simulink model "PneumaticDynamics"  (R2015a)
settings: Solver=ode45  StartTime=0.0  StopTime=120  RelTol=1e-3
InitFcn:
  | %Parameters
  | Patm = 101300; % Pascals
  | Psrc = Patm*2; % Pascals
  | Tamb = 293; %K - ambient temp
  | 
  | %Valve Geometry
  | stroke = 0.1; % m - stroke length
  | x0 = stroke / 2; % m -initial position
  | A = 0.080; % m2 - cap area
  | A_r = 0.02; % m2 - rod area
  | CapDeadSpace = 0.005; % meters - length past stroke
  | RodDeadSpace = 0.005; %meters - length past stroke
  | m = 3; % kg - rod/cap total mass
  | Cd = 0.8; % discharge coefficient
  | 
  | %Thermodynamic Values
  | k = 1.4; % specific heat ratio for air
  | R = 287; % J/Kg/K; % - specific gas constant for air
  | cp = 1012;% J/Kg/K; % - specific heat of air
  | 
  | %Fluid Flow Values
  | Pcr = 0.528; % choked flow ratio
  | C1 = sqrt(2*k/(R*(k-1))); % flow constant
  | C2 = sqrt( k/( R*((k+1)/2)^((k+1)/(k-1)) ) ); % flow cnst.
libraries: simulink x3
settings Model: Creator=Logan  LastModifiedBy=Logan

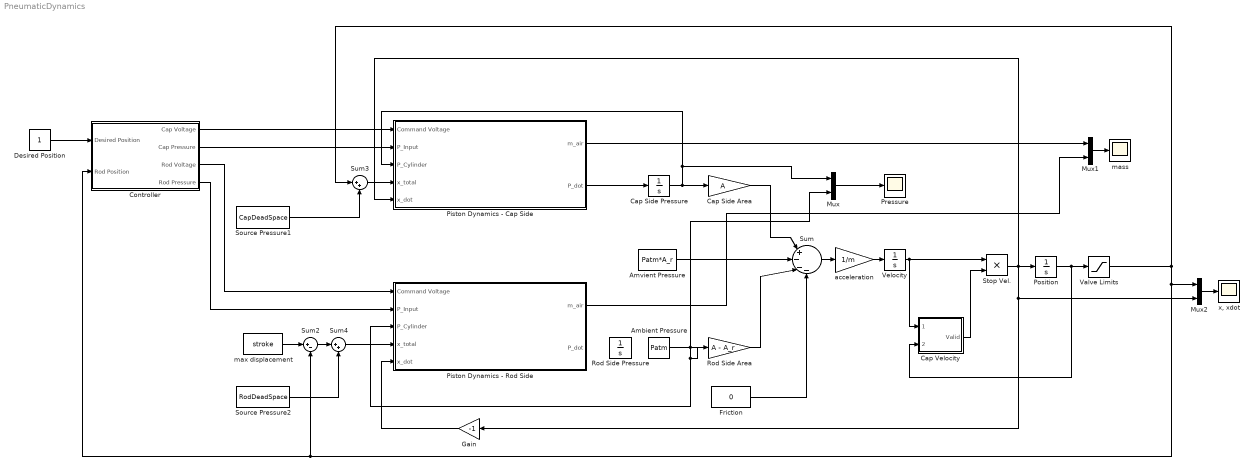
== system PneumaticDynamics ==
  Ambient Pressure : Constant  Value=Patm
  Amvient Pressure : Constant  Value=Patm*A_r
  Cap Side Area : Gain  Gain=A
  Cap Side Pressure : Integrator  InitialCondition=Patm  LimitOutput=on  LowerSaturationLimit=0
  Cap Velocity : Subsystem
  Controller : Subsystem
  Desired Position : Constant
  Friction : Constant  Value=0
  Gain : Gain  Gain=-1
  Mux : Mux  Inputs=2
  Mux1 : Mux  Inputs=2
  Mux2 : Mux  Inputs=2
  Piston Dynamics - Cap Side : Subsystem
  Piston Dynamics - Rod Side : Subsystem
  Position : Integrator  InitialCondition=x0
  Pressure : Scope
      settings: YMin=90000  YMax=155000
  Rod Side Area : Gain  Gain=A - A_r
  Rod Side Pressure : Integrator  InitialCondition=Patm  LimitOutput=on  LowerSaturationLimit=0
  Source Pressure1 : Constant  Value=CapDeadSpace
  Source Pressure2 : Constant  Value=RodDeadSpace
  Stop Vel. : Product
  Sum : Sum  Inputs=|+---
  Sum2 : Sum  Inputs=|+-
  Sum3 : Sum  Inputs=|++
  Sum4 : Sum  Inputs=|++
  Valve Limits : Saturate  UpperLimit=stroke  LowerLimit=0
  Velocity : Integrator
  acceleration : Gain  Gain=1/m
  mass : Scope
      settings: YMin=0.000275  YMax=0.000825
  max displacement : Constant  Value=stroke
  "x, xdot" : Scope
      settings: YMin=-0.0025  YMax=0.0525  SaveName=ScopeData2
  wires:
  Piston Dynamics - Cap Side/2(P_dot) -> Cap Side Pressure/1
  Cap Side Pressure/1 -> Mux/1, Piston Dynamics - Cap Side/3(P_Cylinder), Cap Side Area/1
  Ambient Pressure/1 -> Mux/2, Rod Side Area/1, Piston Dynamics - Rod Side/3(P_Cylinder)
  Cap Side Area/1 -> Sum/1
  Amvient Pressure/1 -> Sum/2
  Rod Side Area/1 -> Sum/3
  Friction/1 -> Sum/4
  Sum/1 -> acceleration/1
  acceleration/1 -> Velocity/1
  Position/1 -> Cap Velocity/2(Position), Valve Limits/1
  max displacement/1 -> Sum2/1
  Source Pressure1/1 -> Sum3/2
  Sum2/1 -> Sum4/1
  Sum4/1 -> Piston Dynamics - Rod Side/4(x_total)
  Source Pressure2/1 -> Sum4/2
  Sum3/1 -> Piston Dynamics - Cap Side/4(x_total)
  Valve Limits/1 -> Sum3/1, Controller/2(Rod Position), Sum2/2, Mux2/1
  Mux/1 -> Pressure/1
  Mux1/1 -> mass/1
  Piston Dynamics - Cap Side/1(m_air) -> Mux1/1
  Piston Dynamics - Rod Side/1(m_air) -> Mux1/2
  Mux2/1 -> "x, xdot"/1
  Stop Vel./1 -> Mux2/2, Gain/1, Position/1, Piston Dynamics - Cap Side/5(x_dot)
  Cap Velocity/1(Valid) -> Stop Vel./2
  Velocity/1 -> Stop Vel./1, Cap Velocity/1(Velocity)
  Desired Position/1 -> Controller/1(Desired Position)
  Controller/1(Cap Voltage) -> Piston Dynamics - Cap Side/1(Command Voltage)
  Controller/2(Cap Pressure) -> Piston Dynamics - Cap Side/2(P_Input)
  Controller/3(Rod Voltage) -> Piston Dynamics - Rod Side/1(Command Voltage)
  Controller/4(Rod Pressure) -> Piston Dynamics - Rod Side/2(P_Input)
  Gain/1 -> Piston Dynamics - Rod Side/5(x_dot)

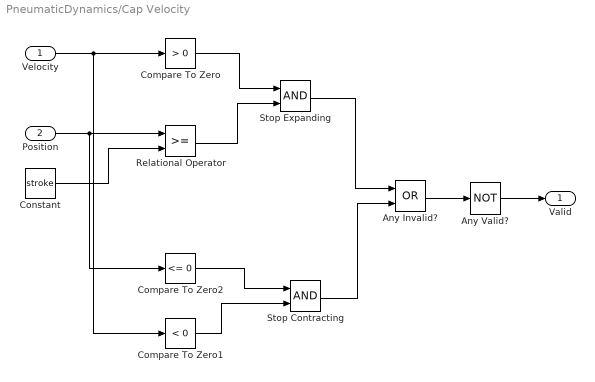
== system PneumaticDynamics/Cap Velocity ==
  Velocity : Inport
  Position : Inport  Port=2
  Any Invalid? : Logic  Operator=OR  AllPortsSameDT=off  OutDataTypeStr=boolean
  Any Valid? : Logic  Operator=NOT  AllPortsSameDT=off  OutDataTypeStr=boolean
  Compare To Zero : simulink/Logic and Bit Operations/Compare To Zero  relop=>  OutDataTypeStr=boolean
  Compare To Zero1 : simulink/Logic and Bit Operations/Compare To Zero  relop=<  OutDataTypeStr=boolean
  Compare To Zero2 : simulink/Logic and Bit Operations/Compare To Zero  relop=<=  OutDataTypeStr=boolean
  Constant : Constant  Value=stroke
  Relational Operator : RelationalOperator  OutDataTypeStr=boolean
  Stop Expanding : Logic  AllPortsSameDT=off  OutDataTypeStr=boolean
  Stop Contracting : Logic  AllPortsSameDT=off  OutDataTypeStr=boolean
  Valid : Outport
  wires:
  Position/1 -> Compare To Zero2/1, Relational Operator/1
  Constant/1 -> Relational Operator/2
  Velocity/1 -> Compare To Zero1/1, Compare To Zero/1
  Compare To Zero/1 -> Stop Expanding/1
  Relational Operator/1 -> Stop Expanding/2
  Compare To Zero2/1 -> Stop Contracting/1
  Compare To Zero1/1 -> Stop Contracting/2
  Stop Expanding/1 -> Any Invalid?/1
  Stop Contracting/1 -> Any Invalid?/2
  Any Invalid?/1 -> Any Valid?/1
  Any Valid?/1 -> Valid/1

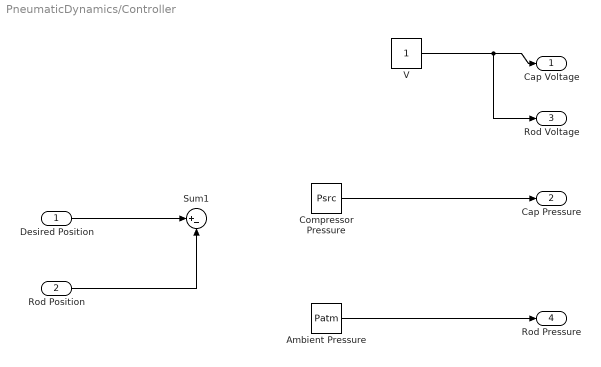
== system PneumaticDynamics/Controller ==
  Desired Position : Inport
  Rod Position : Inport  Port=2
  Ambient Pressure : Constant  Value=Patm
  Compressor Pressure : Constant  Value=Psrc
  Sum1 : Sum  Inputs=|+-
  V : Constant
  Cap Voltage : Outport
  Cap Pressure : Outport  Port=2
  Rod Voltage : Outport  Port=3
  Rod Pressure : Outport  Port=4
  wires:
  Rod Position/1 -> Sum1/2
  Desired Position/1 -> Sum1/1
  Compressor Pressure/1 -> Cap Pressure/1
  V/1 -> Rod Voltage/1, Cap Voltage/1
  Ambient Pressure/1 -> Rod Pressure/1

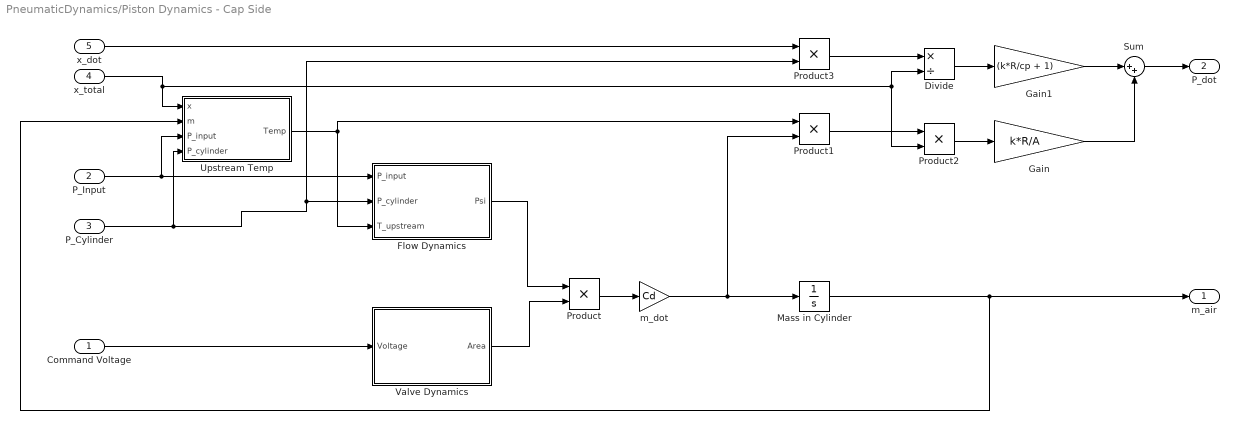
== system PneumaticDynamics/Piston Dynamics - Cap Side ==
  Command Voltage : Inport
  P_Input : Inport  Port=2
  P_Cylinder : Inport  Port=3
  x_total : Inport  Port=4
  x_dot : Inport  Port=5
  Divide : Product  Inputs=*/
  Flow Dynamics : Subsystem
  Gain : Gain  Gain=k*R/A
  Gain1 : Gain  Gain=(k*R/cp + 1)
  Mass in Cylinder : Integrator  InitialCondition=Patm*(x0*A)/R/Tamb
  Product{,1..3} (4 alike) : Product
  Sum : Sum  Inputs=|++
  Upstream Temp : Subsystem
  Valve Dynamics : Subsystem
  m_dot : Gain  Gain=Cd
  m_air : Outport
  P_dot : Outport  Port=2
  wires:
  Product1/1 -> Product2/1
  Product2/1 -> Gain/1
  m_dot/1 -> Mass in Cylinder/1, Product1/2
  Mass in Cylinder/1 -> m_air/1, Upstream Temp/2(m)
  Command Voltage/1 -> Valve Dynamics/1(Voltage)
  P_Input/1 -> Flow Dynamics/1(P_input), Upstream Temp/3(P_input)
  Product3/1 -> Divide/1
  Gain1/1 -> Sum/1
  Product/1 -> m_dot/1
  Divide/1 -> Gain1/1
  x_total/1 -> Product2/2, Divide/2, Upstream Temp/1(x)
  Gain/1 -> Sum/2
  x_dot/1 -> Product3/1
  Flow Dynamics/1(Psi) -> Product/1
  Valve Dynamics/1(Area) -> Product/2
  P_Cylinder/1 -> Flow Dynamics/2(P_cylinder), Product3/2, Upstream Temp/4(P_cylinder)
  Sum/1 -> P_dot/1
  Upstream Temp/1(Temp) -> Flow Dynamics/3(T_upstream), Product1/1

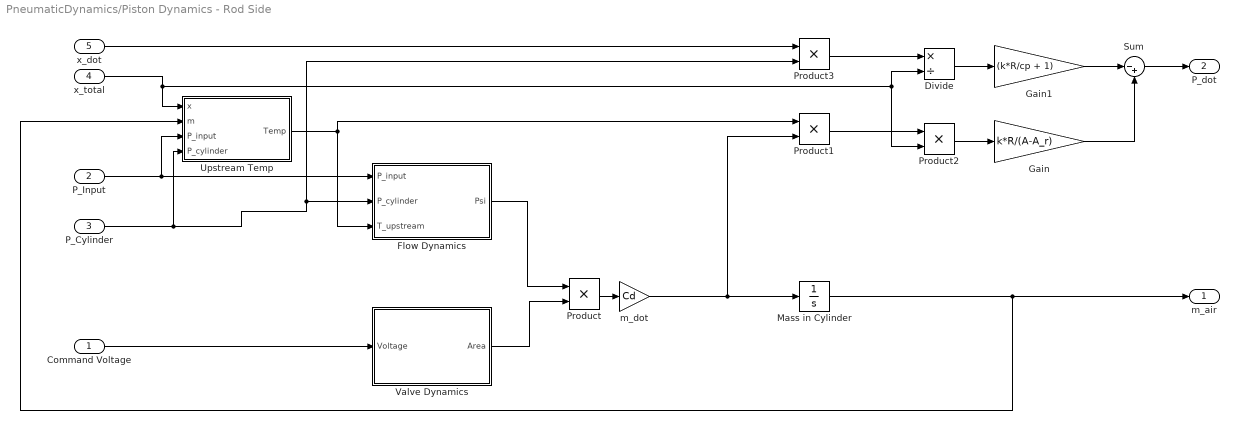
== system PneumaticDynamics/Piston Dynamics - Rod Side ==
  Command Voltage : Inport
  P_Input : Inport  Port=2
  P_Cylinder : Inport  Port=3
  x_total : Inport  Port=4
  x_dot : Inport  Port=5
  Divide : Product  Inputs=*/
  Flow Dynamics : Subsystem
  Gain : Gain  Gain=k*R/(A-A_r)
  Gain1 : Gain  Gain=(k*R/cp + 1)
  Mass in Cylinder : Integrator  InitialCondition=Patm*(x0*(A-A_r))/R/Tamb
  Product{,1..3} (4 alike) : Product
  Sum : Sum  Inputs=|-+
  Upstream Temp : Subsystem
  Valve Dynamics : Subsystem
  m_dot : Gain  Gain=Cd
  m_air : Outport
  P_dot : Outport  Port=2
  wires:
  Product1/1 -> Product2/1
  Product2/1 -> Gain/1
  m_dot/1 -> Mass in Cylinder/1, Product1/2
  Mass in Cylinder/1 -> Upstream Temp/2(m), m_air/1
  Command Voltage/1 -> Valve Dynamics/1(Voltage)
  P_Input/1 -> Flow Dynamics/1(P_input), Upstream Temp/3(P_input)
  Product3/1 -> Divide/1
  Gain1/1 -> Sum/1
  Product/1 -> m_dot/1
  Divide/1 -> Gain1/1
  x_total/1 -> Product2/2, Divide/2, Upstream Temp/1(x)
  Gain/1 -> Sum/2
  x_dot/1 -> Product3/1
  Flow Dynamics/1(Psi) -> Product/1
  Valve Dynamics/1(Area) -> Product/2
  P_Cylinder/1 -> Flow Dynamics/2(P_cylinder), Product3/2, Upstream Temp/4(P_cylinder)
  Sum/1 -> P_dot/1
  Upstream Temp/1(Temp) -> Flow Dynamics/3(T_upstream), Product1/1

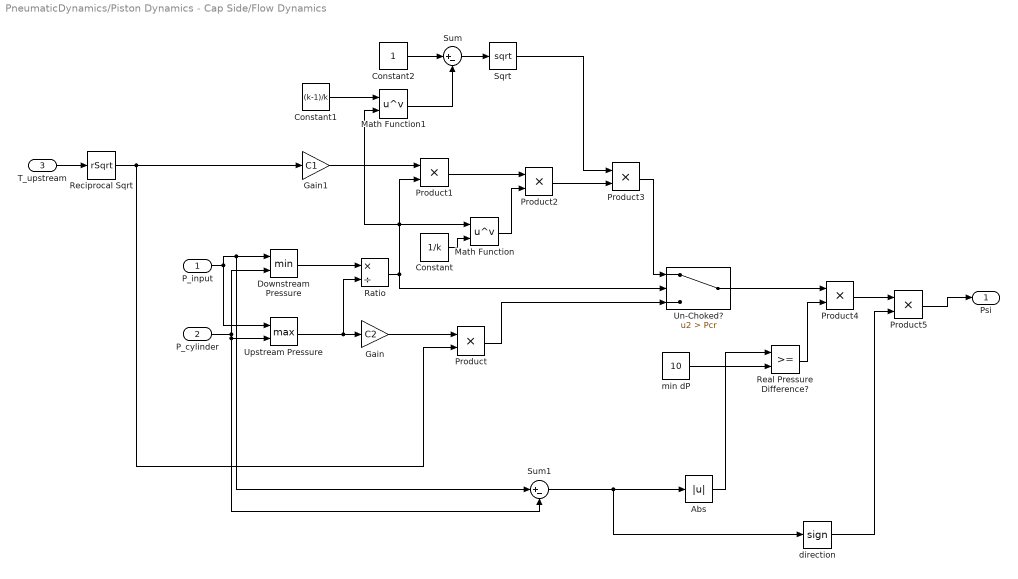
== system PneumaticDynamics/Piston Dynamics - Cap Side/Flow Dynamics ==
  P_input : Inport
  P_cylinder : Inport  Port=2
  T_upstream : Inport  Port=3
  Abs : Abs
  Constant : Constant  Value=1/k
  Constant1 : Constant  Value=(k-1)/k
  Constant2 : Constant
  Downstream Pressure : MinMax  Inputs=2
  Gain : Gain  Gain=C2
  Gain1 : Gain  Gain=C1
  Math Function : Math  Operator=pow  SaturateOnIntegerOverflow=on
  Math Function1 : Math  Operator=pow  SaturateOnIntegerOverflow=on
  Product{,1..5} (6 alike) : Product
  Ratio : Product  Inputs=*/
  Real Pressure Difference? : RelationalOperator  OutDataTypeStr=boolean  ZeroCross=off
  Reciprocal Sqrt : Sqrt  Operator=rSqrt  SaturateOnIntegerOverflow=on
  Sqrt : Sqrt  SaturateOnIntegerOverflow=on
  Sum : Sum  Inputs=|+-
  Sum1 : Sum  Inputs=|+-
  Un-Choked? : Switch  Criteria=u2 > Threshold  Threshold=Pcr  ZeroCross=off
  Upstream Pressure : MinMax  Function=max  Inputs=2
  direction : Signum
  min dP : Constant  Value=10
  Psi : Outport
  wires:
  P_input/1 -> Sum1/1, Downstream Pressure/1, Upstream Pressure/1
  P_cylinder/1 -> Downstream Pressure/2, Sum1/2, Upstream Pressure/2
  Ratio/1 -> Un-Choked?/2, Math Function1/2, Math Function/1, Product1/2
  T_upstream/1 -> Reciprocal Sqrt/1
  Gain/1 -> Product/1
  Reciprocal Sqrt/1 -> Gain1/1, Product/2
  Product/1 -> Un-Choked?/3
  Gain1/1 -> Product1/1
  Product1/1 -> Product2/1
  Constant/1 -> Math Function/2
  Math Function/1 -> Product2/2
  Constant2/1 -> Sum/1
  Math Function1/1 -> Sum/2
  Sum/1 -> Sqrt/1
  Product2/1 -> Product3/2
  Sqrt/1 -> Product3/1
  Constant1/1 -> Math Function1/1
  Product3/1 -> Un-Choked?/1
  Downstream Pressure/1 -> Ratio/1
  Upstream Pressure/1 -> Ratio/2, Gain/1
  Un-Choked?/1 -> Product4/1
  Sum1/1 -> direction/1, Abs/1
  Real Pressure Difference?/1 -> Product4/2
  Abs/1 -> Real Pressure Difference?/1
  min dP/1 -> Real Pressure Difference?/2
  Product4/1 -> Product5/1
  Product5/1 -> Psi/1
  direction/1 -> Product5/2

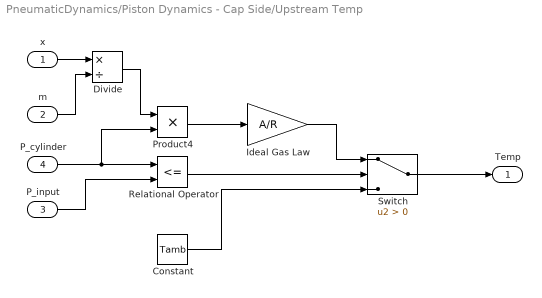
== system PneumaticDynamics/Piston Dynamics - Cap Side/Upstream Temp ==
  x : Inport
  m : Inport  Port=2
  P_input : Inport  Port=3
  P_cylinder : Inport  Port=4
  Constant : Constant  Value=Tamb
  Divide : Product  Inputs=*/
  Ideal Gas Law : Gain  Gain=A/R
  Product4 : Product
  Relational Operator : RelationalOperator  Operator=<=  OutDataTypeStr=boolean
  Switch : Switch  Criteria=u2 > Threshold
  Temp : Outport
  wires:
  Product4/1 -> Ideal Gas Law/1
  Relational Operator/1 -> Switch/2
  Constant/1 -> Switch/3
  P_cylinder/1 -> Product4/2, Relational Operator/1
  P_input/1 -> Relational Operator/2
  Ideal Gas Law/1 -> Switch/1
  Switch/1 -> Temp/1
  Divide/1 -> Product4/1
  x/1 -> Divide/1
  m/1 -> Divide/2

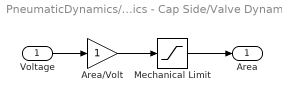
== system PneumaticDynamics/Piston Dynamics - Cap Side/Valve Dynamics ==
  Voltage : Inport
  Area/Volt : Gain
  Mechanical Limit : Saturate  UpperLimit=1  LowerLimit=0
  Area : Outport
  wires:
  Voltage/1 -> Area/Volt/1
  Area/Volt/1 -> Mechanical Limit/1
  Mechanical Limit/1 -> Area/1

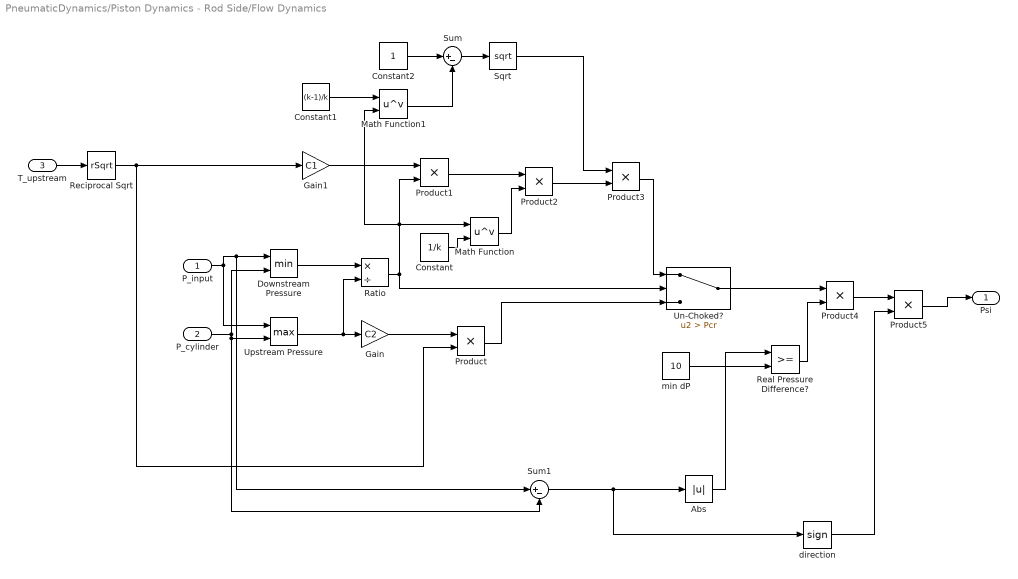
== system PneumaticDynamics/Piston Dynamics - Rod Side/Flow Dynamics ==
  P_input : Inport
  P_cylinder : Inport  Port=2
  T_upstream : Inport  Port=3
  Abs : Abs
  Constant : Constant  Value=1/k
  Constant1 : Constant  Value=(k-1)/k
  Constant2 : Constant
  Downstream Pressure : MinMax  Inputs=2
  Gain : Gain  Gain=C2
  Gain1 : Gain  Gain=C1
  Math Function : Math  Operator=pow  SaturateOnIntegerOverflow=on
  Math Function1 : Math  Operator=pow  SaturateOnIntegerOverflow=on
  Product{,1..5} (6 alike) : Product
  Ratio : Product  Inputs=*/
  Real Pressure Difference? : RelationalOperator  OutDataTypeStr=boolean  ZeroCross=off
  Reciprocal Sqrt : Sqrt  Operator=rSqrt  SaturateOnIntegerOverflow=on
  Sqrt : Sqrt  SaturateOnIntegerOverflow=on
  Sum : Sum  Inputs=|+-
  Sum1 : Sum  Inputs=|+-
  Un-Choked? : Switch  Criteria=u2 > Threshold  Threshold=Pcr  ZeroCross=off
  Upstream Pressure : MinMax  Function=max  Inputs=2
  direction : Signum
  min dP : Constant  Value=10
  Psi : Outport
  wires:
  P_input/1 -> Sum1/1, Downstream Pressure/1, Upstream Pressure/1
  P_cylinder/1 -> Downstream Pressure/2, Sum1/2, Upstream Pressure/2
  Ratio/1 -> Un-Choked?/2, Math Function1/2, Math Function/1, Product1/2
  T_upstream/1 -> Reciprocal Sqrt/1
  Gain/1 -> Product/1
  Reciprocal Sqrt/1 -> Gain1/1, Product/2
  Product/1 -> Un-Choked?/3
  Gain1/1 -> Product1/1
  Product1/1 -> Product2/1
  Constant/1 -> Math Function/2
  Math Function/1 -> Product2/2
  Constant2/1 -> Sum/1
  Math Function1/1 -> Sum/2
  Sum/1 -> Sqrt/1
  Product2/1 -> Product3/2
  Sqrt/1 -> Product3/1
  Constant1/1 -> Math Function1/1
  Product3/1 -> Un-Choked?/1
  Downstream Pressure/1 -> Ratio/1
  Upstream Pressure/1 -> Ratio/2, Gain/1
  Un-Choked?/1 -> Product4/1
  Sum1/1 -> direction/1, Abs/1
  Real Pressure Difference?/1 -> Product4/2
  Abs/1 -> Real Pressure Difference?/1
  min dP/1 -> Real Pressure Difference?/2
  Product4/1 -> Product5/1
  Product5/1 -> Psi/1
  direction/1 -> Product5/2

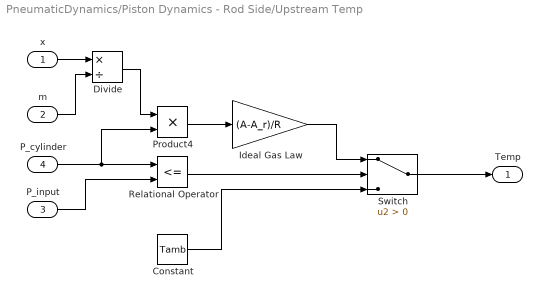
== system PneumaticDynamics/Piston Dynamics - Rod Side/Upstream Temp ==
  x : Inport
  m : Inport  Port=2
  P_input : Inport  Port=3
  P_cylinder : Inport  Port=4
  Constant : Constant  Value=Tamb
  Divide : Product  Inputs=*/
  Ideal Gas Law : Gain  Gain=(A-A_r)/R
  Product4 : Product
  Relational Operator : RelationalOperator  Operator=<=  OutDataTypeStr=boolean
  Switch : Switch  Criteria=u2 > Threshold
  Temp : Outport
  wires:
  Product4/1 -> Ideal Gas Law/1
  Relational Operator/1 -> Switch/2
  Constant/1 -> Switch/3
  P_cylinder/1 -> Product4/2, Relational Operator/1
  P_input/1 -> Relational Operator/2
  Ideal Gas Law/1 -> Switch/1
  Switch/1 -> Temp/1
  Divide/1 -> Product4/1
  x/1 -> Divide/1
  m/1 -> Divide/2

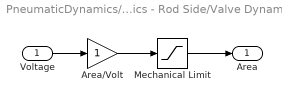
== system PneumaticDynamics/Piston Dynamics - Rod Side/Valve Dynamics ==
  Voltage : Inport
  Area/Volt : Gain
  Mechanical Limit : Saturate  UpperLimit=1  LowerLimit=0
  Area : Outport
  wires:
  Voltage/1 -> Area/Volt/1
  Area/Volt/1 -> Mechanical Limit/1
  Mechanical Limit/1 -> Area/1
